simulink library "tqd"  (R2021b)
settings: Solver=VariableStepAuto  StartTime=0.0  StopTime=10.0  RelTol=1e-3
undefined symbols (not defined in the file or in its folder): ATQD_AccelLimitInRange_X_rpm, ATQD_AccelLimitInRange_Y_Nm, ATQD_AccelLimitOvrKi_X_Nm, ATQD_AccelLimitOvrKp_X_Nm, ATQD_BOSMapD_X_rpm, ATQD_BOSMapD_Y_pct, ATQD_BOSMapR_X_rpm, ATQD_BOSMapR_Y_pct, ATQD_HVBCurrSmooth_X_A, ATQD_LHMTqMapDLC_X_rpm, ATQD_LHMTqMapDLC_Y_pct, ATQD_LHMTqMapRLC_X_rpm, ATQD_LHMTqMapRLC_Y_pct, ATQD_NormalMapDLC_X_rpm, ATQD_NormalMapDLC_Y_pct, ATQD_NormalTqDecSR_X_rpm, ATQD_NormalTqDecSR_Y_Nm, ATQD_NormalTqIncSR_X_rpm, ATQD_NormalTqIncSR_Y_Nm, ATQD_OPDMapRLC_X_rpm, ATQD_OPDMapRLC_Y_pct, ATQD_RollRegTorReq_X_rpm, ATQD_RollRegTorReq_Y_enum, ATQD_VehSpdLimitInRange_X_rpm, ATQD_VehSpdLimitInRange_Y_Nm, ATQD_VehSpdLimitOvrKi_X_Nm, ATQD_VehSpdLimitOvrKp_X_Nm, EIGHT_INT, ENUM_BRAKEPEDAL_PRESSED, ENUM_BRAKEPEDAL_RELEASED, ENUM_COMBOKEY_DOWN, ENUM_COMBOKEY_M1, ENUM_COMBOKEY_M2, ENUM_COMBOKEY_NONE, ENUM_COMBOKEY_RKNEE, ENUM_COMBOKEY_STOPLV, ENUM_COMBOKEY_UP, ENUM_CP2VKNEEREQ_REQUEST, ENUM_CP2VNLVREQ_LEVEL1, ENUM_CP2VNLVREQ_LEVEL2, ENUM_CP2VNLVREQ_LOWER, ENUM_CP2VNLVREQ_STOPLV, ENUM_CP2VNLVREQ_UPPER, ENUM_CREEPIND_DISABLE, ENUM_CREEPIND_READY, ENUM_CREEPIND_RUNNING, ENUM_CREEPIND_WARNING, ENUM_DRIVELINERELEASE_RELEASE, ENUM_EBSTORQUERWQ_LIMIT, ENUM_EBSTORQUERWQ_TORQUE, ENUM_ECPVCUDRM_CONFORT, ENUM_ECPVCUDRM_ECO, ENUM_ECPVCUDRM_NORMAL, ENUM_ECPVCUDRM_NOTAVAILABLE, ENUM_EMTqModeDrvBrk_Accel, ENUM_EMTqModeDrvBrk_Brake, ENUM_EMTqModeDrvBrk_Coast, ENUM_ETC2ACTDRIVEDIR_BACKWARD, ENUM_ETC2ACTDRIVEDIR_FORWARD, ENUM_ETC2ACTDRIVEDIR_STILL ... (+341)
libraries: simulink x109, hcu_lib x67
(part 2 of 13)

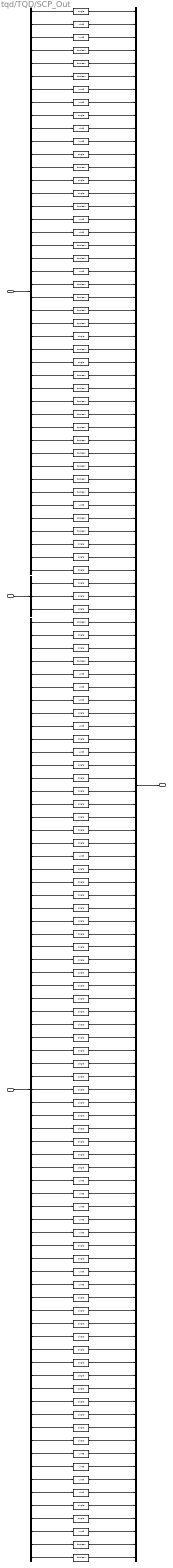
== system tqd/TQD/SCP_Out ==
  BInpConvert_outputs : Inport
  BMain_outputs : Inport  Port=2
  BOutpConvert_outputs : Inport  Port=3
  Bus Creator : BusCreator  Inputs=120  OutDataTypeStr=Bus: BTQD_outputs  NonVirtualBus=on
  Bus Selector1 : BusSelector  OutputSignals=VTQD_PedalMapTq_Nm,VTQD_GearActualPosn_enum,VTQD_TMRotateDirectionReq_enum,VTQD_ParkingPawlPwrOn_flg,VTQD_ParkingPawlEnable_flg,VTQD_DRTransfer_flg,VTQD_TqSource_enum,VTQD_VCUMCUCtrlMdTQD_enum,VTQD_CreepSpdReq_rpm,VTQD_CreepIND_enum,VTQD_ActTUpAIND_enum,VTQD_RollRegTorReq_Nm,VTQD_RollingRegenEnable_flg,VTQD_VCUMCUDemHiPosVal_rpm,VTQD_VehAcclLimitTG_mps2,VTQD_TorqLimDoorOpn_flg,VTQD_VCUEBSHHSw_enum,VTQD_VCUEBSRd4BR_enum,VTQD_ParkingProtectWarning_flg,VTQD_ParkingProtectAction_flg,VTQD_ActDriveMode_enum,VTQD_VCU4PweLmtInd_flg,VTQD_GearFlashIndDis_flg,VTQD_GearFlashInd_flg,VTQD_SpdLimSta_flg,VTQD_EngModeEnDetTime_s,VTQD_EngModeEnDetEnd_flg,VTQD_EngModeDisDetTime_s,VTQD_EngModeDisDetEnd_flg,VTQD_LVchrgSvrMode_flg,VTQD_ActFRDoorOPSta_flg,VTQD_ActMDDoorOPSta_flg,VTQD_ActTDDoorOPSta_flg,VTQD_Function1Off_flg,VTQD_Function2Off_flg,VTQD_Function3Off_flg,VTQD_Function4Off_flg,VTQD_Function5Off_flg,VTQD_FunctionOffSta_enum,VTQD_ComboKeyEn_flg,VTQD_ComboKeyPreEn_flg,VTQD_VehSpdLimitTG_kph,VTQD_VCUTMVehSpd_kph,VTQD_VCUVehSpd_kph
  Bus Selector2 : BusSelector  OutputSignals=VTQD_DriverTqDem_Nm,VTQD_AfterAvailableTqDemRr_Nm,VTQD_TMTqReq_Nm
  Bus Selector3 : BusSelector  OutputSignals=VTQD_TqReductEnable_flg,VTQD_ADASDriverDemWhTq_Nm,VTQD_RealWhTq_Nm,VTQD_VCUBCMBuzzReq_flg,VTQD_VCUEBSHBSw_enum,VTQD_EVCU1ActDrvMode_enum,VTQD_EVCU1WheelSlipdet_enum,VTQD_EVCU1EMotorSpd_rpm,VTQD_EVCU1EMotorOvrerSpd_enum,VTQD_EVCU1EMotorPerformance_pct,VTQD_EVCU1EBrakeTorqLow_enum,VTQD_EVCU2MaxTorqAvail_pct,VTQD_EVCU2MinTorqAvail_pct,VTQD_EEC3NFricPercTorq_pct,VTQD_EEC3EMPressLoss_pct,VTQD_ETC2ActDriveDirect_enum,VTQD_RC1PctTrqP4_pct,VTQD_RC1PctTrqPekTrqP5_pct,VTQD_EMRC1EMTquModeDrvBrk_enum,VTQD_EMRC1ActEMpTrq_pct,VTQD_EMRC1ActEMOutSftSpd_rpm,VTQD_EMRC1ActEMpTrqHrls_pct,VTQD_EMRC1ActMaxAvaEMRecpTrq_pct,VTQD_EC1EMSpdIdleP1_rpm,VTQD_EC1PercTorqIdleP1_pct,VTQD_EC1EMSpdIdleP2_rpm,VTQD_EC1PercTorqIdleP2_pct,VTQD_EC1EMSpdIdleP3_rpm,VTQD_EC1PercTorqIdleP3_pct,VTQD_EC1EMSpdIdleP4_rpm,VTQD_EC1PercTorqIdleP4_pct,VTQD_EC1PercTorqIdleP5_pct,VTQD_EC1EMSpdIdleP5_rpm,VTQD_EC1EMRefTorq_Nm,VTQD_EC1EMMaxMEngOvrSP7_rpm,VTQD_EC1EMMaxMOvrTmt_s,VTQD_EC1EMReqSpdCtrlLoLmt_rpm,VTQD_EC1EMReqTrqCtrlLoLmt_pct,VTQD_EC1EMReqSpdCtrlUpLmt_rpm,VTQD_EC1EMReqTrqCtrlUpLmt_pct,VTQD_EC1EMExtRSCtrlUpLmt_rpm,VTQD_EC1EMMomOfInertia_kgpm2,VTQD_EC1EMDefTrqLmt_rpm,VTQD_EC1EMSupVarRTSC1MSG_cnt,VTQD_EC1EMSupTSC1CtrlPG1_cnt,VTQD_EC1EMSupTSC1CtrlPG3_cnt,VTQD_EC1EMSupTSC1CtrlPG2_cnt,VTQD_EC1EMSupTSC1CtrlPG4_cnt,VTQD_EC1EMSpdHdleP6_rpm,VTQD_EC1EMGainEndSpdGvn_gain,VTQD_RC1RetType_enum,VTQD_RC1RetLocat_enum,VTQD_RC1RetCtrlMth_enum,VTQD_RC1RetSpdIdleP1_rpm,VTQD_RC1PctTrqIdleP1_pct,VTQD_RC1MaxRetSpdP2_rpm,VTQD_RC1RetSpdP2_pct,VTQD_RC1MaxRetSpdP3_rpm,VTQD_RC1PctTrqP3_pct,VTQD_RC1RefRetTrq_Nm,VTQD_RC1RetSpdPekTrqP5_Nm,VTQD_RC1RetSpdP4_rpm,VTQD_VCUMCUDemLoNegVal_rpm,VTQD_VCUMCUDemSpd_rpm,VTQD_VCUMCUGearSta_enum,VTQD_TUpAIND_enum,VTQD_ETC1ShiftrPgs_enum,VTQD_EVCU1RecuperHighSta_enum,VTQD_EMRC1DrvDemEMRtapTrq_pct,VTQD_EMRC1RetSelNonEng_pct,VTQD_EMRC1SACtrlDev_cnt,VTQD_VCUMCUHandBrk_flg,VTQD_VCUMCUFootBrk_flg
  Data Type Conversion{,8,11,13..14,26,28,42..44,46..47,52,54,56..62,64..87,93..94,97..108,112..115,119} (64 alike) : DataTypeConversion  OutDataTypeStr=single
  Data Type Conversion{1..2,6..7,9..10,16..17,20,24,39,49..51,53,55,63,88..92,95..96,109..111,116} (28 alike) : DataTypeConversion  OutDataTypeStr=uint8
  Data Type Conversion{3..5,12,15,18..19,21..23,25,27,29..38,40..41,45,48,117..118} (28 alike) : DataTypeConversion  OutDataTypeStr=boolean
  BTQD_outputs : Outport  OutDataTypeStr=Bus:BTQD_outputs
  wires:
  Bus Selector3/7 -> Data Type Conversion51/1  "<VTQD_EVCU1WheelSlipdet_enum>"
  Bus Selector3/30 -> Data Type Conversion74/1  "<VTQD_EC1EMSpdIdleP4_rpm>"
  Bus Selector3/45 -> Data Type Conversion89/1  "<VTQD_EC1EMSupTSC1CtrlPG1_cnt>"
  Bus Selector3/19 -> Data Type Conversion63/1  "<VTQD_EMRC1EMTquModeDrvBrk_enum>"
  Bus Selector1/2 -> Data Type Conversion1/1  "<VTQD_GearActualPosn_enum>"
  Bus Selector2/3 -> Data Type Conversion44/1  "<VTQD_TMTqReq_Nm>"
  Bus Selector3/18 -> Data Type Conversion62/1  "<VTQD_RC1PctTrqPekTrqP5_pct>"
  Bus Selector3/44 -> Data Type Conversion88/1  "<VTQD_EC1EMSupVarRTSC1MSG_cnt>"
  Bus Selector3/31 -> Data Type Conversion75/1  "<VTQD_EC1PercTorqIdleP4_pct>"
  Bus Selector3/15 -> Data Type Conversion59/1  "<VTQD_EEC3EMPressLoss_pct>"
  Bus Selector3/66 -> Data Type Conversion110/1  "<VTQD_TUpAIND_enum>"
  Bus Selector1/13 -> Data Type Conversion12/1  "<VTQD_RollingRegenEnable_flg>"
  Bus Selector1/31 -> Data Type Conversion31/1  "<VTQD_ActFRDoorOPSta_flg>"
  Bus Selector1/10 -> Data Type Conversion9/1  "<VTQD_CreepIND_enum>"
  Bus Selector3/28 -> Data Type Conversion72/1  "<VTQD_EC1EMSpdIdleP3_rpm>"
  Bus Selector1/36 -> Data Type Conversion36/1  "<VTQD_Function3Off_flg>"
  Bus Selector3/33 -> Data Type Conversion77/1  "<VTQD_EC1EMSpdIdleP5_rpm>"
  Bus Selector3/23 -> Data Type Conversion67/1  "<VTQD_EMRC1ActMaxAvaEMRecpTrq_pct>"
  BOutpConvert_outputs/1 -> Bus Selector3/1
  Bus Selector1/33 -> Data Type Conversion33/1  "<VTQD_ActTDDoorOPSta_flg>"
  Bus Selector3/47 -> Data Type Conversion91/1  "<VTQD_EC1EMSupTSC1CtrlPG2_cnt>"
  Bus Selector1/24 -> Data Type Conversion23/1  "<VTQD_GearFlashInd_flg>"
  Bus Selector3/4 -> Data Type Conversion48/1  "<VTQD_VCUBCMBuzzReq_flg>"
  Bus Selector3/24 -> Data Type Conversion68/1  "<VTQD_EC1EMSpdIdleP1_rpm>"
  Bus Selector1/18 -> Data Type Conversion17/1  "<VTQD_VCUEBSRd4BR_enum>"
  BInpConvert_outputs/1 -> Bus Selector1/1
  Bus Selector1/8 -> Data Type Conversion7/1  "<VTQD_VCUMCUCtrlMdTQD_enum>"
  Bus Selector3/21 -> Data Type Conversion65/1  "<VTQD_EMRC1ActEMOutSftSpd_rpm>"
  Bus Selector1/22 -> Data Type Conversion21/1  "<VTQD_VCU4PweLmtInd_flg>"
  Bus Selector3/29 -> Data Type Conversion73/1  "<VTQD_EC1PercTorqIdleP3_pct>"
  Bus Selector3/3 -> Data Type Conversion47/1  "<VTQD_RealWhTq_Nm>"
  Bus Selector1/9 -> Data Type Conversion8/1  "<VTQD_CreepSpdReq_rpm>"
  Bus Selector3/51 -> Data Type Conversion95/1  "<VTQD_RC1RetType_enum>"
  Bus Selector1/26 -> Data Type Conversion26/1  "<VTQD_EngModeEnDetTime_s>"
  Bus Selector1/29 -> Data Type Conversion29/1  "<VTQD_EngModeDisDetEnd_flg>"
  Bus Selector3/6 -> Data Type Conversion50/1  "<VTQD_EVCU1ActDrvMode_enum>"
  Bus Selector1/17 -> Data Type Conversion16/1  "<VTQD_VCUEBSHHSw_enum>"
  Bus Selector3/9 -> Data Type Conversion53/1  "<VTQD_EVCU1EMotorOvrerSpd_enum>"
  Bus Selector3/26 -> Data Type Conversion70/1  "<VTQD_EC1EMSpdIdleP2_rpm>"
  Bus Selector3/25 -> Data Type Conversion69/1  "<VTQD_EC1PercTorqIdleP1_pct>"
  Bus Selector1/23 -> Data Type Conversion22/1  "<VTQD_GearFlashIndDis_flg>"
  Bus Selector3/22 -> Data Type Conversion66/1  "<VTQD_EMRC1ActEMpTrqHrls_pct>"
  Bus Selector3/68 -> Data Type Conversion111/1  "<VTQD_EVCU1RecuperHighSta_enum>"
  Bus Selector3/5 -> Data Type Conversion49/1  "<VTQD_VCUEBSHBSw_enum>"
  Bus Selector1/5 -> Data Type Conversion4/1  "<VTQD_ParkingPawlEnable_flg>"
  Bus Selector3/65 -> Data Type Conversion109/1  "<VTQD_VCUMCUGearSta_enum>"
  Bus Selector3/14 -> Data Type Conversion58/1  "<VTQD_EEC3NFricPercTorq_pct>"
  Bus Selector1/28 -> Data Type Conversion28/1  "<VTQD_EngModeDisDetTime_s>"
  Bus Selector3/50 -> Data Type Conversion94/1  "<VTQD_EC1EMGainEndSpdGvn_gain>"
  Bus Selector3/16 -> Data Type Conversion60/1  "<VTQD_ETC2ActDriveDirect_enum>"
  Bus Selector1/3 -> Data Type Conversion2/1  "<VTQD_TMRotateDirectionReq_enum>"
  Bus Selector3/36 -> Data Type Conversion80/1  "<VTQD_EC1EMMaxMOvrTmt_s>"
  Bus Selector1/7 -> Data Type Conversion6/1  "<VTQD_TqSource_enum>"
  Bus Selector3/27 -> Data Type Conversion71/1  "<VTQD_EC1PercTorqIdleP2_pct>"
  Bus Selector3/34 -> Data Type Conversion78/1  "<VTQD_EC1EMRefTorq_Nm>"
  Bus Selector1/6 -> Data Type Conversion5/1  "<VTQD_DRTransfer_flg>"
  Bus Selector1/21 -> Data Type Conversion20/1  "<VTQD_ActDriveMode_enum>"
  Bus Selector3/32 -> Data Type Conversion76/1  "<VTQD_EC1PercTorqIdleP5_pct>"
  Bus Selector3/48 -> Data Type Conversion92/1  "<VTQD_EC1EMSupTSC1CtrlPG4_cnt>"
  Bus Selector1/42 -> Data Type Conversion112/1  "<VTQD_VehSpdLimitTG_kph>"
  Bus Selector1/37 -> Data Type Conversion37/1  "<VTQD_Function4Off_flg>"
  Bus Selector1/32 -> Data Type Conversion32/1  "<VTQD_ActMDDoorOPSta_flg>"
  Bus Selector3/2 -> Data Type Conversion46/1  "<VTQD_ADASDriverDemWhTq_Nm>"
  Bus Selector1/39 -> Data Type Conversion39/1  "<VTQD_FunctionOffSta_enum>"
  Bus Selector1/20 -> Data Type Conversion19/1  "<VTQD_ParkingProtectAction_flg>"
  Bus Selector1/38 -> Data Type Conversion38/1  "<VTQD_Function5Off_flg>"
  Bus Selector3/52 -> Data Type Conversion96/1  "<VTQD_RC1RetLocat_enum>"
  Bus Selector1/30 -> Data Type Conversion30/1  "<VTQD_LVchrgSvrMode_flg>"
  Bus Selector1/11 -> Data Type Conversion10/1  "<VTQD_ActTUpAIND_enum>"
  Bus Selector3/43 -> Data Type Conversion87/1  "<VTQD_EC1EMDefTrqLmt_rpm>"
  Bus Selector3/37 -> Data Type Conversion81/1  "<VTQD_EC1EMReqSpdCtrlLoLmt_rpm>"
  Bus Selector3/11 -> Data Type Conversion55/1  "<VTQD_EVCU1EBrakeTorqLow_enum>"
  Bus Selector3/55 -> Data Type Conversion99/1  "<VTQD_RC1PctTrqIdleP1_pct>"
  Bus Selector1/12 -> Data Type Conversion11/1  "<VTQD_RollRegTorReq_Nm>"
  Bus Selector3/39 -> Data Type Conversion83/1  "<VTQD_EC1EMReqSpdCtrlUpLmt_rpm>"
  Bus Selector1/19 -> Data Type Conversion18/1  "<VTQD_ParkingProtectWarning_flg>"
  Bus Selector3/42 -> Data Type Conversion86/1  "<VTQD_EC1EMMomOfInertia_kgpm2>"
  Bus Selector1/34 -> Data Type Conversion34/1  "<VTQD_Function1Off_flg>"
  Bus Selector3/59 -> Data Type Conversion103/1  "<VTQD_RC1PctTrqP3_pct>"
  Bus Selector1/35 -> Data Type Conversion35/1  "<VTQD_Function2Off_flg>"
  Bus Selector1/27 -> Data Type Conversion27/1  "<VTQD_EngModeEnDetEnd_flg>"
  Bus Selector3/17 -> Data Type Conversion61/1  "<VTQD_RC1PctTrqP4_pct>"
  Bus Selector3/20 -> Data Type Conversion64/1  "<VTQD_EMRC1ActEMpTrq_pct>"
  Bus Selector1/25 -> Data Type Conversion25/1  "<VTQD_SpdLimSta_flg>"
  Bus Selector3/35 -> Data Type Conversion79/1  "<VTQD_EC1EMMaxMEngOvrSP7_rpm>"
  Bus Selector3/49 -> Data Type Conversion93/1  "<VTQD_EC1EMSpdHdleP6_rpm>"
  Bus Selector3/58 -> Data Type Conversion102/1  "<VTQD_RC1MaxRetSpdP3_rpm>"
  Bus Selector2/1 -> Data Type Conversion42/1  "<VTQD_DriverTqDem_Nm>"
  Bus Selector3/38 -> Data Type Conversion82/1  "<VTQD_EC1EMReqTrqCtrlLoLmt_pct>"
  Bus Selector3/8 -> Data Type Conversion52/1  "<VTQD_EVCU1EMotorSpd_rpm>"
  Bus Selector3/12 -> Data Type Conversion56/1  "<VTQD_EVCU2MaxTorqAvail_pct>"
  Bus Selector3/57 -> Data Type Conversion101/1  "<VTQD_RC1RetSpdP2_pct>"
  Bus Selector3/60 -> Data Type Conversion104/1  "<VTQD_RC1RefRetTrq_Nm>"
  Bus Selector3/13 -> Data Type Conversion57/1  "<VTQD_EVCU2MinTorqAvail_pct>"
  Bus Selector3/62 -> Data Type Conversion106/1  "<VTQD_RC1RetSpdP4_rpm>"
  Bus Selector1/4 -> Data Type Conversion3/1  "<VTQD_ParkingPawlPwrOn_flg>"
  Bus Selector1/1 -> Data Type Conversion/1  "<VTQD_PedalMapTq_Nm>"
  Bus Selector3/56 -> Data Type Conversion100/1  "<VTQD_RC1MaxRetSpdP2_rpm>"
  Bus Selector1/41 -> Data Type Conversion41/1  "<VTQD_ComboKeyPreEn_flg>"
  BMain_outputs/1 -> Bus Selector2/1
  Bus Selector3/67 -> Data Type Conversion24/1  "<VTQD_ETC1ShiftrPgs_enum>"
  Bus Selector1/15 -> Data Type Conversion14/1  "<VTQD_VehAcclLimitTG_mps2>"
  Bus Creator/1 -> BTQD_outputs/1  "Bus:BTQD_outputs"
  Bus Selector3/1 -> Data Type Conversion45/1  "<VTQD_TqReductEnable_flg>"
  Bus Selector1/40 -> Data Type Conversion40/1  "<VTQD_ComboKeyEn_flg>"
  Bus Selector3/46 -> Data Type Conversion90/1  "<VTQD_EC1EMSupTSC1CtrlPG3_cnt>"
  Bus Selector3/63 -> Data Type Conversion107/1  "<VTQD_VCUMCUDemLoNegVal_rpm>"
  Bus Selector3/64 -> Data Type Conversion108/1  "<VTQD_VCUMCUDemSpd_rpm>"
  Bus Selector3/40 -> Data Type Conversion84/1  "<VTQD_EC1EMReqTrqCtrlUpLmt_pct>"
  Bus Selector1/16 -> Data Type Conversion15/1  "<VTQD_TorqLimDoorOpn_flg>"
  Bus Selector1/14 -> Data Type Conversion13/1  "<VTQD_VCUMCUDemHiPosVal_rpm>"
  Bus Selector2/2 -> Data Type Conversion43/1  "<VTQD_AfterAvailableTqDemRr_Nm>"
  Bus Selector3/41 -> Data Type Conversion85/1  "<VTQD_EC1EMExtRSCtrlUpLmt_rpm>"
  Bus Selector3/61 -> Data Type Conversion105/1  "<VTQD_RC1RetSpdPekTrqP5_Nm>"
  Bus Selector3/54 -> Data Type Conversion98/1  "<VTQD_RC1RetSpdIdleP1_rpm>"
  Bus Selector3/10 -> Data Type Conversion54/1  "<VTQD_EVCU1EMotorPerformance_pct>"
  Bus Selector3/53 -> Data Type Conversion97/1  "<VTQD_RC1RetCtrlMth_enum>"
  Bus Selector1/43 -> Data Type Conversion113/1  "<VTQD_VCUTMVehSpd_kph>"
  Data Type Conversion/1 -> Bus Creator/1  "VTQD_PedalMapTq_Nm"
  Data Type Conversion1/1 -> Bus Creator/2  "VTQD_GearActualPosn_enum"
  Data Type Conversion2/1 -> Bus Creator/3  "VTQD_TMRotateDirectionReq_enum"
  Data Type Conversion3/1 -> Bus Creator/4  "VTQD_ParkingPawlPwrOn_flg"
  Data Type Conversion4/1 -> Bus Creator/5  "VTQD_ParkingPawlEnable_flg"
  Data Type Conversion5/1 -> Bus Creator/6  "VTQD_DRTransfer_flg"
  Data Type Conversion6/1 -> Bus Creator/7  "VTQD_TqSource_enum"
  Data Type Conversion7/1 -> Bus Creator/8  "VTQD_VCUMCUCtrlMdTQD_enum"
  Data Type Conversion8/1 -> Bus Creator/9  "VTQD_CreepSpdReq_rpm"
  Data Type Conversion9/1 -> Bus Creator/10  "VTQD_CreepIND_enum"
  Data Type Conversion10/1 -> Bus Creator/11  "VTQD_ActTUpAIND_enum"
  Data Type Conversion11/1 -> Bus Creator/12  "VTQD_RollRegTorReq_Nm"
  Data Type Conversion12/1 -> Bus Creator/13  "VTQD_RollingRegenEnable_flg"
  Data Type Conversion13/1 -> Bus Creator/14  "VTQD_VCUMCUDemHiPosVal_rpm"
  Data Type Conversion14/1 -> Bus Creator/15  "VTQD_VehAcclLimitTG_mps2"
  Data Type Conversion15/1 -> Bus Creator/16  "VTQD_TorqLimDoorOpn_flg"
  Data Type Conversion16/1 -> Bus Creator/17  "VTQD_VCUEBSHHSw_enum"
  Data Type Conversion17/1 -> Bus Creator/18  "VTQD_VCUEBSRd4BR_enum"
  Data Type Conversion18/1 -> Bus Creator/19  "VTQD_ParkingProtectWarning_flg"
  Data Type Conversion19/1 -> Bus Creator/20  "VTQD_ParkingProtectAction_flg"
  Data Type Conversion20/1 -> Bus Creator/21  "VTQD_ActDriveMode_enum"
  Data Type Conversion21/1 -> Bus Creator/22  "VTQD_VCU4PweLmtInd_flg"
  Data Type Conversion22/1 -> Bus Creator/23  "VTQD_GearFlashIndDis_flg"
  Data Type Conversion23/1 -> Bus Creator/24  "VTQD_GearFlashInd_flg"
  Data Type Conversion25/1 -> Bus Creator/25  "VTQD_SpdLimSta_flg"
  Data Type Conversion26/1 -> Bus Creator/26  "VTQD_EngModeEnDetTime_s"
  Data Type Conversion27/1 -> Bus Creator/27  "VTQD_EngModeEnDetEnd_flg"
  Data Type Conversion28/1 -> Bus Creator/28  "VTQD_EngModeDisDetTime_s"
  Data Type Conversion29/1 -> Bus Creator/29  "VTQD_EngModeDisDetEnd_flg"
  Data Type Conversion30/1 -> Bus Creator/30  "VTQD_LVchrgSvrMode_flg"
  Data Type Conversion31/1 -> Bus Creator/31  "VTQD_ActFRDoorOPSta_flg"
  Data Type Conversion32/1 -> Bus Creator/32  "VTQD_ActMDDoorOPSta_flg"
  Data Type Conversion33/1 -> Bus Creator/33  "VTQD_ActTDDoorOPSta_flg"
  Data Type Conversion34/1 -> Bus Creator/34  "VTQD_Function1Off_flg"
  Data Type Conversion35/1 -> Bus Creator/35  "VTQD_Function2Off_flg"
  Data Type Conversion36/1 -> Bus Creator/36  "VTQD_Function3Off_flg"
  Data Type Conversion37/1 -> Bus Creator/37  "VTQD_Function4Off_flg"
  Data Type Conversion38/1 -> Bus Creator/38  "VTQD_Function5Off_flg"
  Data Type Conversion39/1 -> Bus Creator/39  "VTQD_FunctionOffSta_enum"
  Data Type Conversion40/1 -> Bus Creator/40  "VTQD_ComboKeyEn_flg"
  Data Type Conversion41/1 -> Bus Creator/41  "VTQD_ComboKeyPreEn_flg"
  Data Type Conversion112/1 -> Bus Creator/42  "VTQD_VehSpdLimitTG_kph"
  Data Type Conversion113/1 -> Bus Creator/43  "VTQD_VCUTMVehSpd_kph"
  Bus Selector3/69 -> Data Type Conversion114/1  "<VTQD_EMRC1DrvDemEMRtapTrq_pct>"
  Bus Selector3/70 -> Data Type Conversion115/1  "<VTQD_EMRC1RetSelNonEng_pct>"
  Bus Selector3/71 -> Data Type Conversion116/1  "<VTQD_EMRC1SACtrlDev_cnt>"
  Bus Selector3/72 -> Data Type Conversion117/1  "<VTQD_VCUMCUHandBrk_flg>"
  Bus Selector3/73 -> Data Type Conversion118/1  "<VTQD_VCUMCUFootBrk_flg>"
  Bus Selector1/44 -> Data Type Conversion119/1  "<VTQD_VCUVehSpd_kph>"
  Data Type Conversion45/1 -> Bus Creator/48  "VTQD_TqReductEnable_flg"
  Data Type Conversion44/1 -> Bus Creator/47  "VTQD_TMTqReq_Nm"
  Data Type Conversion43/1 -> Bus Creator/46  "VTQD_AfterAvailableTqDemRr_Nm"
  Data Type Conversion42/1 -> Bus Creator/45  "VTQD_DriverTqDem_Nm"
  Data Type Conversion119/1 -> Bus Creator/44  "VTQD_VCUVehSpd_kph"
  Data Type Conversion51/1 -> Bus Creator/54  "VTQD_EVCU1WheelSlipdet_enum"
  Data Type Conversion50/1 -> Bus Creator/53  "VTQD_EVCU1ActDrvMode_enum"
  Data Type Conversion52/1 -> Bus Creator/55  "VTQD_EVCU1EMotorSpd_rpm"
  Data Type Conversion49/1 -> Bus Creator/52  "VTQD_VCUEBSHBSw_enum"
  Data Type Conversion53/1 -> Bus Creator/56  "VTQD_EVCU1EMotorOvrerSpd_enum"
  Data Type Conversion48/1 -> Bus Creator/51  "VTQD_VCUBCMBuzzReq_flg"
  Data Type Conversion54/1 -> Bus Creator/57  "VTQD_EVCU1EMotorPerformance_pct"
  Data Type Conversion47/1 -> Bus Creator/50  "VTQD_RealWhTq_Nm"
  Data Type Conversion46/1 -> Bus Creator/49  "VTQD_ADASDriverDemWhTq_Nm"
  Data Type Conversion55/1 -> Bus Creator/58  "VTQD_EVCU1EBrakeTorqLow_enum"
  Data Type Conversion56/1 -> Bus Creator/59  "VTQD_EVCU2MaxTorqAvail_pct"
  Data Type Conversion57/1 -> Bus Creator/60  "VTQD_EVCU2MinTorqAvail_pct"
  Data Type Conversion58/1 -> Bus Creator/61  "VTQD_EEC3NFricPercTorq_pct"
  Data Type Conversion59/1 -> Bus Creator/62  "VTQD_EEC3EMPressLoss_pct"
  Data Type Conversion60/1 -> Bus Creator/63  "VTQD_ETC2ActDriveDirect_enum"
  Data Type Conversion61/1 -> Bus Creator/64  "VTQD_RC1PctTrqP4_pct"
  Data Type Conversion62/1 -> Bus Creator/65  "VTQD_RC1PctTrqPekTrqP5_pct"
  Data Type Conversion63/1 -> Bus Creator/66  "VTQD_EMRC1EMTquModeDrvBrk_enum"
  Data Type Conversion64/1 -> Bus Creator/67  "VTQD_EMRC1ActEMpTrq_pct"
  Data Type Conversion65/1 -> Bus Creator/68  "VTQD_EMRC1ActEMOutSftSpd_rpm"
  Data Type Conversion66/1 -> Bus Creator/69  "VTQD_EMRC1ActEMpTrqHrls_pct"
  Data Type Conversion67/1 -> Bus Creator/70  "VTQD_EMRC1ActMaxAvaEMRecpTrq_pct"
  Data Type Conversion68/1 -> Bus Creator/71  "VTQD_EC1EMSpdIdleP1_rpm"
  Data Type Conversion69/1 -> Bus Creator/72  "VTQD_EC1PercTorqIdleP1_pct"
  Data Type Conversion70/1 -> Bus Creator/73  "VTQD_EC1EMSpdIdleP2_rpm"
  Data Type Conversion71/1 -> Bus Creator/74  "VTQD_EC1PercTorqIdleP2_pct"
  Data Type Conversion72/1 -> Bus Creator/75  "VTQD_EC1EMSpdIdleP3_rpm"
  Data Type Conversion73/1 -> Bus Creator/76  "VTQD_EC1PercTorqIdleP3_pct"
  Data Type Conversion74/1 -> Bus Creator/77  "VTQD_EC1EMSpdIdleP4_rpm"
  Data Type Conversion75/1 -> Bus Creator/78  "VTQD_EC1PercTorqIdleP4_pct"
  Data Type Conversion76/1 -> Bus Creator/79  "VTQD_EC1PercTorqIdleP5_pct"
  Data Type Conversion77/1 -> Bus Creator/80  "VTQD_EC1EMSpdIdleP5_rpm"
  Data Type Conversion78/1 -> Bus Creator/81  "VTQD_EC1EMRefTorq_Nm"
  Data Type Conversion79/1 -> Bus Creator/82  "VTQD_EC1EMMaxMEngOvrSP7_rpm"
  Data Type Conversion80/1 -> Bus Creator/83  "VTQD_EC1EMMaxMOvrTmt_s"
  Data Type Conversion81/1 -> Bus Creator/84  "VTQD_EC1EMReqSpdCtrlLoLmt_rpm"
  Data Type Conversion82/1 -> Bus Creator/85  "VTQD_EC1EMReqTrqCtrlLoLmt_pct"
  Data Type Conversion83/1 -> Bus Creator/86  "VTQD_EC1EMReqSpdCtrlUpLmt_rpm"
  Data Type Conversion84/1 -> Bus Creator/87  "VTQD_EC1EMReqTrqCtrlUpLmt_pct"
  Data Type Conversion85/1 -> Bus Creator/88  "VTQD_EC1EMExtRSCtrlUpLmt_rpm"
  Data Type Conversion86/1 -> Bus Creator/89  "VTQD_EC1EMMomOfInertia_kgpm2"
  Data Type Conversion87/1 -> Bus Creator/90  "VTQD_EC1EMDefTrqLmt_rpm"
  Data Type Conversion88/1 -> Bus Creator/91  "VTQD_EC1EMSupVarRTSC1MSG_cnt"
  Data Type Conversion89/1 -> Bus Creator/92  "VTQD_EC1EMSupTSC1CtrlPG1_cnt"
  Data Type Conversion90/1 -> Bus Creator/93  "VTQD_EC1EMSupTSC1CtrlPG3_cnt"
  Data Type Conversion91/1 -> Bus Creator/94  "VTQD_EC1EMSupTSC1CtrlPG2_cnt"
  Data Type Conversion92/1 -> Bus Creator/95  "VTQD_EC1EMSupTSC1CtrlPG4_cnt"
  Data Type Conversion93/1 -> Bus Creator/96  "VTQD_EC1EMSpdHdleP6_rpm"
  Data Type Conversion94/1 -> Bus Creator/97  "VTQD_EC1EMGainEndSpdGvn_gain"
  Data Type Conversion95/1 -> Bus Creator/98  "VTQD_RC1RetType_enum"
  Data Type Conversion96/1 -> Bus Creator/99  "VTQD_RC1RetLocat_enum"
  Data Type Conversion97/1 -> Bus Creator/100  "VTQD_RC1RetCtrlMth_enum"
  Data Type Conversion98/1 -> Bus Creator/101  "VTQD_RC1RetSpdIdleP1_rpm"
  Data Type Conversion99/1 -> Bus Creator/102  "VTQD_RC1PctTrqIdleP1_pct"
  Data Type Conversion100/1 -> Bus Creator/103  "VTQD_RC1MaxRetSpdP2_rpm"
  Data Type Conversion101/1 -> Bus Creator/104  "VTQD_RC1RetSpdP2_pct"
  Data Type Conversion102/1 -> Bus Creator/105  "VTQD_RC1MaxRetSpdP3_rpm"
  Data Type Conversion103/1 -> Bus Creator/106  "VTQD_RC1PctTrqP3_pct"
  Data Type Conversion104/1 -> Bus Creator/107  "VTQD_RC1RefRetTrq_Nm"
  Data Type Conversion105/1 -> Bus Creator/108  "VTQD_RC1RetSpdPekTrqP5_Nm"
  Data Type Conversion106/1 -> Bus Creator/109  "VTQD_RC1RetSpdP4_rpm"
  Data Type Conversion107/1 -> Bus Creator/110  "VTQD_VCUMCUDemLoNegVal_rpm"
  Data Type Conversion108/1 -> Bus Creator/111  "VTQD_VCUMCUDemSpd_rpm"
  Data Type Conversion109/1 -> Bus Creator/112  "VTQD_VCUMCUGearSta_enum"
  Data Type Conversion110/1 -> Bus Creator/113  "VTQD_TUpAIND_enum"
  Data Type Conversion24/1 -> Bus Creator/114  "VTQD_ETC1ShiftrPgs_enum"
  Data Type Conversion111/1 -> Bus Creator/115  "VTQD_EVCU1RecuperHighSta_enum"
  Data Type Conversion114/1 -> Bus Creator/116  "VTQD_EMRC1DrvDemEMRtapTrq_pct"
  Data Type Conversion115/1 -> Bus Creator/117  "VTQD_EMRC1RetSelNonEng_pct"
  Data Type Conversion116/1 -> Bus Creator/118  "VTQD_EMRC1SACtrlDev_cnt"
  Data Type Conversion117/1 -> Bus Creator/119  "VTQD_VCUMCUHandBrk_flg"
  Data Type Conversion118/1 -> Bus Creator/120  "VTQD_VCUMCUFootBrk_flg"

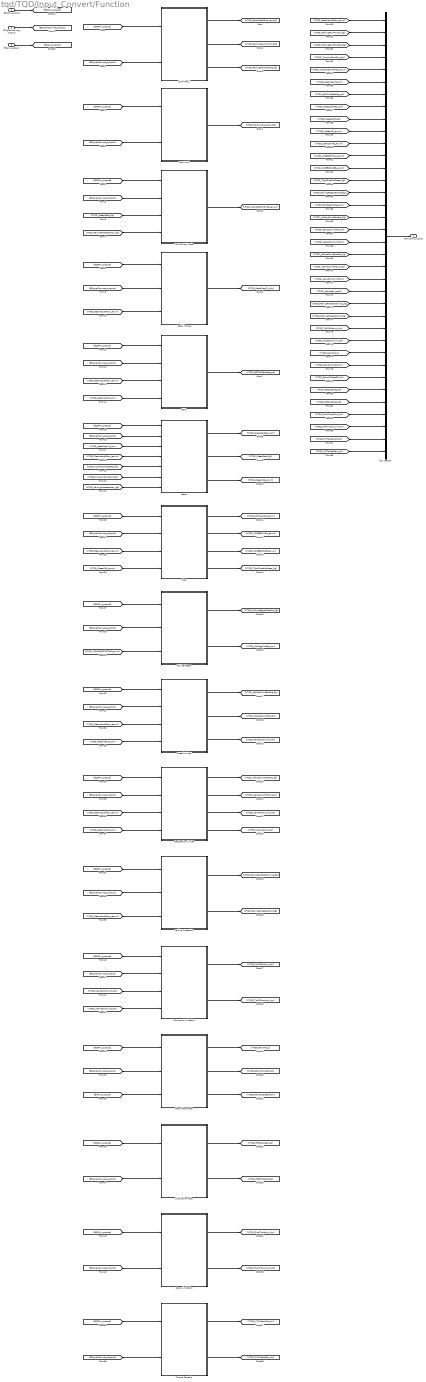
== system tqd/TQD/Input_Convert/Function ==
  BSCPIn_outputs : Inport
  BSignalConvert_outputs : Inport  Port=2
  BMain_outputs : Inport  Port=3
  Acceleration Limiter : Subsystem
      settings: RTWSystemCode=Nonreusable function
  BOS : Subsystem
      settings: RTWSystemCode=Nonreusable function
  Bus Creator : BusCreator  Inputs=36
  Command Limitation : Subsystem
      settings: RTWSystemCode=Nonreusable function
  Creep : Subsystem
      settings: RTWSystemCode=Nonreusable function
  Distribution Rate : Subsystem  TreatAsAtomicUnit=on
      settings: RTWSystemCode=Nonreusable function
  Door Limit : Subsystem
      settings: RTWSystemCode=Nonreusable function
  MCU Control Mode : Subsystem
      settings: RTWSystemCode=Nonreusable function
  Parking Protection : Subsystem
      settings: RTWSystemCode=Nonreusable function
  Pedal Torque : Subsystem
      settings: RTWSystemCode=Nonreusable function
  Ramp Limitation : Subsystem  TreatAsAtomicUnit=on
      settings: RTWSystemCode=Nonreusable function
  Ramp Parameter : Subsystem
      settings: RTWSystemCode=Nonreusable function
  Rolling Regen : Subsystem
      settings: RTWSystemCode=Nonreusable function
  Shift Modul : Subsystem
      settings: RTWSystemCode=Nonreusable function
  Speed Limiter : Subsystem
      settings: RTWSystemCode=Nonreusable function
  TUpA : Subsystem
      settings: RTWSystemCode=Nonreusable function
  Torque Capacity : Subsystem  TreatAsAtomicUnit=on
      settings: RTWSystemCode=Nonreusable function
  BFunction_outputs : Outport
  wires:
  Shift Modul/1(VTQD_GearActualPosn_enum) -> [VTQD_GearActualPosn_enum]
  [VTQD_TqCMDUpLim_Nm] -> Bus Creator/26
  [BSCPIn_outputs] -> Pedal Torque/1(BSCPIn_outputs)
  TUpA/3(VTQD_VCUEBSRd4BR_enum) -> [VTQD_VCUEBSRd4BR_enum]
  TUpA/2(VTQD_VCUEBSHHSw_enum) -> [VTQD_VCUEBSHHSw_enum]
  [VTQD_GearActualPosn_enum] -> BOS/3(VTQD_GearActualPosn_enum)
  [VTQD_GearActualPosn_enum] -> Creep/4(VTQD_GearActualPosn_enum)
  [VTQD_RrEDUSpRat_rat] -> Bus Creator/32
  [VTQD_FinalTrqLowLim_Nm] -> Bus Creator/34
  [BSignalConvert_outputs] -> Ramp Limitation/2(BSignalConvert_outputs)
  Rolling Regen/2(VTQD_RollRegTorReq_Nm) -> [VTQD_RollRegTorReq_Nm]
  [BSCPIn_outputs] -> Shift Modul/1(BSCPIn_outputs)
  [BSCPIn_outputs] -> Door Limit/1(BSCPIn_outputs)
  BSCPIn_outputs/1 -> [BSCPIn_outputs]
  Pedal Torque/1(VTQD_PedalMapTq_Nm) -> [VTQD_PedalMapTq_Nm]
  Shift Modul/3(VTQD_ParkingPawlEnable_flg) -> [VTQD_ParkingPawlEnable_flg]
  BSignalConvert_outputs/1 -> [BSignalConvert_outputs]
  [VTQD_CreepIND_enum] -> TUpA/4(VTQD_CreepIND_enum)
  [VTQD_GearActualPosn_enum] -> TUpA/3(VTQD_GearActualPosn_enum)
  TUpA/1(VTQD_ActTUpAIND_enum) -> [VTQD_ActTUpAIND_enum]
  Door Limit/1(VTQD_TorqLimDoorOpn_flg) -> [VTQD_TorqLimDoorOpn_flg]
  [BSignalConvert_outputs] -> Shift Modul/2(BSignalConvert_outputs)
  [VTQD_GearActualPosn_enum] -> Acceleration Limiter/3(VTQD_GearActualPosn_enum)
  [VTQD_ActTUpAIND_enum] -> Bus Creator/11
  MCU Control Mode/1(VTQD_VCUMCUCtrlMdTQD_enum) -> [VTQD_VCUMCUCtrlMdTQD_enum]
  Speed Limiter/3(VTQD_VehSpdTorLimit_Nm) -> [VTQD_VehSpdTorLimit_Nm]
  [VTQD_ParkingProtectAction_flg] -> MCU Control Mode/4(VTQD_ParkingProtectAction_flg)
  Shift Modul/2(VTQD_ParkingPawlPwrOn_flg) -> [VTQD_ParkingPawlPwrOn_flg]
  Parking Protection/1(VTQD_ParkingProtectWarning_flg) -> [VTQD_ParkingProtectWarning_flg]
  [VTQD_GearActualPosn_enum] -> Pedal Torque/3(VTQD_GearActualPosn_enum)
  [VTQD_PedalMapTq_Nm] -> Acceleration Limiter/4(VTQD_PedalMapTq_Nm)
  Acceleration Limiter/3(VTQD_VehAcclTorLimit_Nm) -> [VTQD_VehAcclTorLimit_Nm]
  [BSignalConvert_outputs] -> MCU Control Mode/2(BSignalConvert_outputs)
  [BSignalConvert_outputs] -> BOS/2(BSignalConvert_outputs)
  Acceleration Limiter/1(VTQD_VehAcclLimitEnable_flg) -> [VTQD_VehAcclLimitEnable_flg]
  [BSignalConvert_outputs] -> Creep/2(BSignalConvert_outputs)
  [VTQD_ParkingProtectAction_flg] -> Bus Creator/25
  [BSCPIn_outputs] -> MCU Control Mode/1(BSCPIn_outputs)
  [BSignalConvert_outputs] -> Acceleration Limiter/2(BSignalConvert_outputs)
  [BSignalConvert_outputs] -> Command Limitation/2(BSignalConvert_outputs)
  BOS/1(VTQD_BOSTqDecRate_pct) -> [VTQD_BOSTqDecRate_pct]
  [BSCPIn_outputs] -> BOS/1(BSCPIn_outputs)
  [VTQD_ParkingPawlEnable_flg] -> Bus Creator/3
  [BSCPIn_outputs] -> Parking Protection/1(BSCPIn_outputs)
  [VTQD_PedalMapTq_Nm] -> Bus Creator/6
  [VTQD_ParkingProtectAction_flg] -> Creep/7(VTQD_ParkingProtectAction_flg)
  [BSCPIn_outputs] -> Rolling Regen/1(BSCPIn_outputs)
  Acceleration Limiter/4(VTQD_VehAccel_mps2) -> [VTQD_VehAccel_mps2]
  [BSCPIn_outputs] -> Creep/1(BSCPIn_outputs)
  [VTQD_TUpADisableCreep_flg] -> Creep/5(VTQD_TUpADisableCreep_flg)
  [VTQD_PedalMapTq_Nm] -> Creep/3(VTQD_PedalMapTq_Nm)
  Creep/1(VTQD_CreepSpdReq_rpm) -> [VTQD_CreepSpdReq_rpm]
  [VTQD_TorqLimDoorOpn_flg] -> Creep/6(VTQD_TorqLimDoorOpn_flg)
  [BSignalConvert_outputs] -> TUpA/2(BSignalConvert_outputs)
  Creep/3(VTQD_CreepIND_enum) -> [VTQD_CreepIND_enum]
  [VTQD_GearActualPosn_enum] -> Parking Protection/3(VTQD_GearActualPosn_enum)
  [BSCPIn_outputs] -> TUpA/1(BSCPIn_outputs)
  [VTQD_CreepStart_flg] -> MCU Control Mode/3(VTQD_CreepStart_flg)
  Distribution Rate/1(VTQD_FrEDUSpRat_rat) -> [VTQD_FrEDUSpRat_rat]
  [BSCPIn_outputs] -> Acceleration Limiter/1(BSCPIn_outputs)
  Creep/2(VTQD_CreepStart_flg) -> [VTQD_CreepStart_flg]
  [BSCPIn_outputs] -> Speed Limiter/1(BSCPIn_outputs)
  [VTQD_PedalMapTq_Nm] -> Speed Limiter/4(VTQD_PedalMapTq_Nm)
  [VTQD_PedalMapTq_Nm] -> BOS/4(VTQD_PedalMapTq_Nm)
  Speed Limiter/1(VTQD_VehSpdLimitEnable_flg) -> [VTQD_VehSpdLimitEnable_flg]
  [BSignalConvert_outputs] -> Rolling Regen/2(BSignalConvert_outputs)
  Speed Limiter/2(VTQD_VehSpdLimitTG_kph) -> [VTQD_VehSpdLimitTG_kph]
  TUpA/4(VTQD_TUpADisableCreep_flg) -> [VTQD_TUpADisableCreep_flg]
  [VTQD_RollRegTorReq_Nm] -> Bus Creator/16
  [VTQD_VehSpdTorLimit_Nm] -> Bus Creator/19
  [VTQD_GearActualPosn_enum] -> Speed Limiter/3(VTQD_GearActualPosn_enum)
  Rolling Regen/1(VTQD_RollingRegenEnable_flg) -> [VTQD_RollingRegenEnable_flg]
  [VTQD_TqCMDLowLim_Nm] -> Bus Creator/27
  Acceleration Limiter/2(VTQD_VehAcclLimitTG_mps2) -> [VTQD_VehAcclLimitTG_mps2]
  [VTQD_VehSpdTorLimit_Nm] -> Command Limitation/3(VTQD_VehSpdTorLimit_Nm)
  [VTQD_VCUMCUCtrlMdTQD_enum] -> Rolling Regen/3(VTQD_VCUMCUCtrlMdTQD_enum)
  [BSignalConvert_outputs] -> Door Limit/2(BSignalConvert_outputs)
  [VTQD_VehAcclTorLimit_Nm] -> Command Limitation/4(VTQD_VehAcclTorLimit_Nm)
  [VTQD_VCUEBSHHSw_enum] -> Bus Creator/12
  Parking Protection/2(VTQD_ParkingProtectAction_flg) -> [VTQD_ParkingProtectAction_flg]
  [BSignalConvert_outputs] -> Pedal Torque/2(BSignalConvert_outputs)
  [BSCPIn_outputs] -> Command Limitation/1(BSCPIn_outputs)
  [BSignalConvert_outputs] -> Parking Protection/2(BSignalConvert_outputs)
  Command Limitation/1(VTQD_TqCMDUpLim_Nm) -> [VTQD_TqCMDUpLim_Nm]
  [BSignalConvert_outputs] -> Speed Limiter/2(BSignalConvert_outputs)
  Command Limitation/2(VTQD_TqCMDLowLim_Nm) -> [VTQD_TqCMDLowLim_Nm]
  [BSCPIn_outputs] -> Ramp Parameter/1(BSCPIn_outputs)
  [BSignalConvert_outputs] -> Ramp Parameter/2(BSignalConvert_outputs)
  [VTQD_RampTqIncSR_Nm] -> Bus Creator/29
  [VTQD_GearActualPosn_enum] -> Bus Creator/1
  [VTQD_VehSpdLimitEnable_flg] -> Bus Creator/17
  [VTQD_RampTqDecSR_Nm] -> Bus Creator/30
  [VTQD_VehAcclLimitTG_mps2] -> Bus Creator/21
  [VTQD_VCUEBSRd4BR_enum] -> Bus Creator/13
  [VTQD_BOSTqDecRate_pct] -> Bus Creator/7
  [VTQD_FinalTrqUpLim_Nm] -> Bus Creator/33
  Ramp Parameter/3(VTQD_RampTqDecSR_Nm) -> [VTQD_RampTqDecSR_Nm]
  [VTQD_VCUMCUCtrlMdTQD_enum] -> Bus Creator/5
  Ramp Parameter/1(VTQD_RampTs_c) -> [VTQD_RampTs_c]
  [VTQD_VehAcclLimitEnable_flg] -> Bus Creator/20
  [VTQD_FrEDUSpRat_rat] -> Bus Creator/31
  Ramp Parameter/2(VTQD_RampTqIncSR_Nm) -> [VTQD_RampTqIncSR_Nm]
  [VTQD_CreepStart_flg] -> Bus Creator/9
  [BSCPIn_outputs] -> Ramp Limitation/1(BSCPIn_outputs)
  [VTQD_TorqLimDoorOpn_flg] -> Bus Creator/4
  [VTQD_RampTs_c] -> Bus Creator/28
  Ramp Limitation/1(VTQD_FinalTrqUpLim_Nm) -> [VTQD_FinalTrqUpLim_Nm]
  Distribution Rate/2(VTQD_RrEDUSpRat_rat) -> [VTQD_RrEDUSpRat_rat]
  [BSCPIn_outputs] -> Distribution Rate/1(BSCPIn_outputs)
  Ramp Limitation/2(VTQD_FinalTrqLowLim_Nm) -> [VTQD_FinalTrqLowLim_Nm]
  [VTQD_ParkingPawlPwrOn_flg] -> Bus Creator/2
  [BSignalConvert_outputs] -> Distribution Rate/2(BSignalConvert_outputs)
  [VTQD_VehSpdLimitTG_kph] -> Bus Creator/18
  [VTQD_VehAccel_mps2] -> Bus Creator/23
  [VTQD_CreepIND_enum] -> Bus Creator/10
  [VTQD_VehAcclTorLimit_Nm] -> Bus Creator/22
  [VTQD_ParkingProtectWarning_flg] -> Bus Creator/24
  [VTQD_CreepSpdReq_rpm] -> Bus Creator/8
  Bus Creator/1 -> BFunction_outputs/1  "BFunction_outputs"
  [VTQD_RollingRegenEnable_flg] -> Bus Creator/15
  [VTQD_TUpADisableCreep_flg] -> Bus Creator/14
  BMain_outputs/1 -> [BMain_outputs]
  [BMain_outputs] -> Ramp Parameter/3(BMain_outputs)
  [BSCPIn_outputs] -> Torque Capacity/1(BSCPIn_outputs)
  [BSignalConvert_outputs] -> Torque Capacity/2(BSignalConvert_outputs)
  Torque Capacity/2(VTQD_TMTqCapGen_Nm) -> [VTQD_TMTqCapGen_Nm]
  Torque Capacity/1(VTQD_TMTqCapMot_Nm) -> [VTQD_TMTqCapMot_Nm]
  [VTQD_TMTqCapMot_Nm] -> Bus Creator/35
  [VTQD_TMTqCapGen_Nm] -> Bus Creator/36
